simulink model "quadcopter_package_delivery"  (R2022a)
settings: Solver=ode23t  StartTime=0.0  StopTime=timespot_spl(end)+4  FixedStep=0.01  MaxStep=1e-2  RelTol=1e-3  AbsTol=1e-3
PostLoadFcn:
  | warning('off','sm:sli:setup:compile:LocalSolverNotSupported')
model workspace (MATLAB code in the model file):
  | load('xy_data_membrane.mat');
undefined symbols (not defined in the file): battery_capacity, filtD_altitude, filtD_attitude, filtD_motor, filtD_position, filtD_yaw, filtM_altitude, filtM_attitude, filtM_position, filtM_yaw, filtSpd_motor, kd_altitude, kd_attitude, kd_motor, kd_position, kd_yaw, ki_altitude, ki_attitude, ki_motor, ki_position, ki_yaw, kp_altitude, kp_attitude, kp_motor, kp_position, kp_yaw, limit_altitude, limit_attitude, limit_motor, limit_yaw, pkgDensity, planedepth, pos2attitude, qd_area, qd_drag, spline_data, spline_yaw, timespot_spl, waypoints, X, Y, Z
libraries: sm_lib x104, nesl_utility x61, fl_lib x21, slpidlib x9, ee_lib x5, quadcopter_library x4
(part 1 of 5)
CloseFcn:
  | try,close(h1_quadcopter_package_delivery),end
  | clear h1_quadcopter_package_delivery
  | try,close(h2_quadcopter_package_delivery),end
  | clear h2_quadcopter_package_delivery
  | try,close(h3_quadcopter_package_delivery),end
  | clear h3_quadcopter_package_delivery
  | try,close(h4_quadcopter_package_delivery),end
  | clear h4_quadcopter_package_delivery
Description:
  | Quadcopter Package Delivery
  | Copyright 2021 The MathWorks, Inc.
settings Model: Creator=tianwang  LastModifiedBy=johnsongash
settings SolverCC: AutoScaleAbsTol=off  AlgebraicLoopSolver=TrustRegion  SolverResetMethod=Robust
settings DataIOCC: MaxDataPoints=10000  ReturnWorkspaceOutputs=off  SignalLoggingName=logsout_quadcopter_package_delivery
settings DebuggingCC: ParameterPrecisionLossMsg=none  UnconnectedInputMsg=warning  UnconnectedOutputMsg=warning  UnconnectedLineMsg=warning  SFMachineParentedDataDiag=warning
settings SFSimCC: CustomCodeUndefinedFunction=UseInterfaceOnly
settings RTWCC: DLArmComputeVersion=19.05
settings SimscapeCC: ExplicitSolverDiagnosticOptions=none  SimscapeLogType=all  SimscapeLogSimulationStatistics=on  SimscapeLogToSDI=on  SimscapeLogName=simlog_quadcopter_package_delivery  SimscapeLogDataHistory=10000
settings DiagnosticsConfigSet: SimMechanicsConflictingReferenceFrames=none  SimMechanicsRigidlyBoundBlock=none
settings ExplorerConfigSet: InternalSimMechanicsExplorerSettings="<ExplorerConfiguration><canonicalview>default</canonicalview><AnimationSetting><BasePlaybackSpeed>1.0</BasePlaybackSpeed><PlaybackSpeedFactor>2.0</PlaybackSpeedFactor></AnimationSetting><TilePanel><TileInfo><Tiles Columns=\"2\" Count=\"4\" Rows=\"2\"><Column Weight=\"0.5664\"/><Column Weight=\"0.4336\"/><Row Weight=\"0.3531\"/><Row Weight=\"0.6469\"/><Tile Height=\"1\" Width=\"1\" X=\"0\" Y=\"0\"/><Tile Height=\"1\" Width=\"1\" X=\"0\" Y=\"1\"/><Tile Height=\"1\" Width=\"1\" X=\"1\" Y=\"0\"/><Tile Height=\"1\" Width=\"1\" X=\"1\" Y=\"1\"/></Tiles></TileInfo><SceneInfo><SceneViewer><BGColor><R>1</R><G>1</G><B>1</B></BGColor><Camera><DoPerspective>off</DoPerspective><Position><X>3.00027489530859626</X><Y>2.64492473252887361</Y><Z>13.644244441979108</Z></Position><Center><X>3.00027489530859626</X><Y>2.64492473252887361</Y><Z>3.00000062058594352</Z></Center><Up><X>0</X><Y>1</Y><Z>-0</Z></Up><ViewLimDist>1</ViewLimDist><YLim>10.5985457420349132</YLim><XLim>33.4261827248793395</XLim></Camera></SceneViewer><SceneViewer><BGColor><R>1</R><G>1</G><B>1</B></BGColor><Camera><DoPerspective>on</DoPerspective><Position><X>5.02017998369651863</X><Y>7.98844218227809488</Y><Z>3.70518563279751856</Z></Position><Center><X>5.02017998369651863</X><Y>7.98844218227809488</Y><Z>2.70518563279751856</Z></Center><Up><X>0</X><Y>1</Y><Z>0</Z></Up><ViewLimDist>1</ViewLimDist><YLim>0.466307658154998583</YLim><XLim>0.796608916014789226</XLim></Camera></SceneViewer><SceneViewer><BGColor><R>1</R><G>1</G><B>1</B></BGColor><Camera><DoPerspective>on</DoPerspective><Position><X>6.5</X><Y>6.5</Y><Z>1</Z></Position><Center><X>5</X><Y>8</Y><Z>0</Z></Center><Up><X>0</X><Y>0</Y><Z>1</Z></Up><ViewLimDist>1</ViewLimDist><YLim>0.466307658154998583</YLim><XLim>1.12272536155780434</XLim></Camera></SceneViewer><SceneViewer><BGColor><R>1</R><G>1</G><B>1</B></BGColor><Camera><DoPerspective>on</DoPerspective><Position><X>5.52017998369651863</X><Y>6.98844218227809488</Y><Z>3.70518563279751856</Z></Position><Center><X>5.1868466503631856</X><Y>7.65510884894476185</Y><Z>3.0385189661308516</Z></Center><Up><X>-0.298142396999971915</X><Y>0.596284793999944052</Y><Z>0.745355992499929787</Z></Up><ViewLimDist>1</ViewLimDist><YLim>0.466307658154998583</YLim><XLim>0.608142904177144006</XLim></Camera></SceneViewer></SceneInfo></TilePanel><MechEditorPanel><Cameras><Camera><Id>Camera1</Id><Value><Name>FixO Top</Name><NativeCamera><PositionTrackingFeature>Quadcopter.Camera.Cam_FixO_Top.R</PositionTrackingFeature><CenterTrackingFeature>Quadcopter.Camera.Cam_FixO_Top.R</CenterTrackingFeature><UpVectorTrackingFeature>Quadcopter.Camera.Cam_FixO_Top.R</UpVectorTrackingFeature><CenterTrackingOrigin>off</CenterTrackingOrigin><CenterTrackingDirection>+X</CenterTrackingDirection><UpVectorTrackingDirection>+Y</UpVectorTrackingDirection></NativeCamera></Value></Camera><Camera><Id>Camera2</Id><Value><Name>FixO L</Name><NativeCamera><PositionTrackingFeature>Quadcopter.Camera.Cam_FixO_L.R</PositionTrackingFeature><CenterTrackingFeature>Quadcopter.Camera.Cam_FixO_L.R</CenterTrackingFeature><UpVectorTrackingFeature>Quadcopter.Camera.Cam_FixO_L.R</UpVectorTrackingFeature><CenterTrackingOrigin>off</CenterTrackingOrigin><CenterTrackingDirection>+X</CenterTrackingDirection><UpVectorTrackingDirection>+Z</UpVectorTrackingDirection></NativeCamera></Value></Camera><Camera><Id>Camera3</Id><Value><Name>FixO F</Name><NativeCamera><PositionTrackingFeature>Quadcopter.Camera.Cam_FixO_F.R</PositionTrackingFeature><CenterTrackingFeature>Quadcopter.Camera.Cam_FixO_F.R</CenterTrackingFeature><UpVectorTrackingFeature>Quadcopter.Camera.Cam_FixO_F.R</UpVectorTrackingFeature><CenterTrackingOrigin>off</CenterTrackingOrigin><CenterTrackingDirection>+X</CenterTrackingDirection><UpVectorTrackingDirection>+Z</UpVectorTrackingDirection></NativeCamera></Value></Camera><Camera><Id>Camera4</Id><Value><Name>FixO UFL</Name><NativeCamera><PositionTrackingFeature>Quadcopter.Camera.Cam_FixO_UFL.R</PositionTrackingFeature><CenterTrackingFeature>Quadcopter.Camera.Cam_FixO_UFL.R</CenterTrackingFeature><UpVectorTrackingFeature>Quadcopter.Camera.Cam_FixO_UFL.R</UpVectorTrackingFeature><CenterTrackingOrigin>off</CenterTrackingOrigin><CenterTrackingDirection>+X</CenterTrackingDirection><UpVectorTrackingDirection>+Z</UpVectorTrackingDirection></NativeCamera></Value></Camera><Camera><Id>Camera5</Id><Value><Name>Track_Target</Name><NativeCamera><PositionTrackingFeature>Quadcopter.Camera.Cam_Target.R</PositionTrackingFeature><CenterTrackingFeature>Quadcopter.Camera.Transform_Target.F</CenterTrackingFeature><UpVectorTrackingFeature>Quadcopter.Camera.Transform_Target.F</UpVectorTrackingFeature><CenterTrackingOrigin>on</CenterTrackingOrigin><UpVectorTrackingDirection>+Z</UpVectorTrackingDirection></NativeCamera></Value></Camera><Camera><Id>Camera6</Id><Value><Name>Track Body Forward</Name><NativeCamera><PositionTrackingFeature>Quadcopter.Body.Body.Cam_Body_Front.R</PositionTrackingFeature><CenterTrackingFeature>Quadcopter.Body.Body.Cam_Body_Front.R</CenterTrackingFeature><UpVectorTrackingFeature>Quadcopter.Body.Body.Cam_Body_Front.R</UpVectorTrackingFeature><CenterTrackingOrigin>off</CenterTrackingOrigin><CenterTrackingDirection>+X</CenterTrackingDirection><UpVectorTrackingDirection>+Z</UpVectorTrackingDirection></NativeCamera></Value></Camera></Cameras><GfxPanelCameraMap><MapElement CameraMLId=\"Camera1\" GfxPanelIndex=\"1\"/><MapElement CameraMLId=\"Camera5\" GfxPanelIndex=\"2\"/><MapElement CameraMLId=\"Camera4\" GfxPanelIndex=\"3\"/></GfxPanelCameraMap><VideoCreator><PlaybackSpeedRatio>1.0</PlaybackSpeedRatio><FrameRate>60</FrameRate><VideoFormat>MPEG-4</VideoFormat><FrameSize>[1920 1080]</FrameSize></VideoCreator></MechEditorPanel></ExplorerConfiguration>"

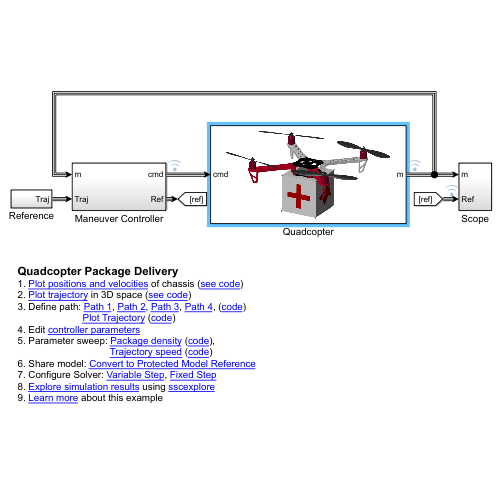
[thumbnail: Simulink's stored preview of the top-level diagram]
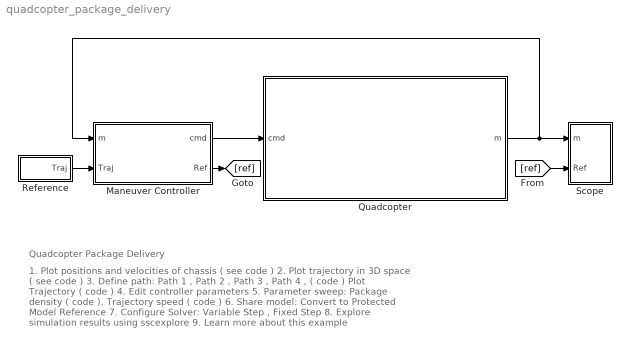
== system quadcopter_package_delivery ==
  note: Quadcopter Package Delivery
  note: 1. Plot positions and velocities of chassis ( see code )
      | 2. Plot trajectory in 3D space ( see code )
      | 3. Define path: Path 1 , Path 2 , Path 3 , Path 4 , ( code )
      | Plot Trajectory ( code )
      | 4. Edit controller parameters
      | 5. Parameter sweep: Package density ( code ),
      | Trajectory speed ( code )
      | 6. Share model: Convert to Protected Model Reference
      | 7. Configure Solver: Variable Step , Fixed Step
      | 8. Explore simulation results using sscexplore
      | 9. Learn more about this example
  Maneuver Controller : Subsystem
  Quadcopter : Subsystem
      mask Display: image('quadcopter_body_arms_load.png');
  Reference : Subsystem
  Scope : Subsystem
  wires:
  Maneuver Controller/1(cmd) -> Quadcopter/1(cmd)
  Quadcopter/1(m) -> Scope/1(m), Maneuver Controller/1(m)
  Reference/1(Traj) -> Maneuver Controller/2(Traj)
  [ref] -> Scope/2(Ref)
  Maneuver Controller/2(Ref) -> [ref]

== system quadcopter_package_delivery/Maneuver Controller ==
  In Bus Element13 : Inport  PortName=m
  In Bus Element3 : Inport  Port=2  PortName=Traj
  Altitude and YPR Control : Subsystem  mask{attitude_filtM=filtM_attitude, attitude_kp=kp_attitude, attitude_ki=ki_attitude, attitude_kd=kd_attitude, attitude_f=filtD_attitude, attitude_limit=limit_attitude, yaw_filtM=filtM_yaw, yaw_kp=kp_yaw, yaw_ki=ki_yaw, yaw_kd=kd_yaw, yaw_f=filtD_yaw, yaw_limit=limit_yaw, altitude_filtM=filtM_altitude, altitude_kp=kp_altitude, altitude_ki=ki_altitude, altitude_kd=kd_altitude, altitude_f=filtD_altitude, altitude_limit=limit_altitude}
      mask prompts: attitude_filtM "Filter Measurement (s)"; attitude_kp "Kp"; attitude_ki "Ki"; attitude_kd "Kd"; attitude_f "Derivative Filter Coefficient"; attitude_limit "Limit (m/s)"; yaw_filtM "Filter Measurement (s)"; yaw_kp "Kp"; yaw_ki "Ki"; yaw_kd "Kd"; yaw_f "Derivative Filter Coefficient"; yaw_limit "Limit (m/s)"; altitude_filtM "Filter Measurement (s)"; altitude_kp "Kp"; altitude_ki "Ki"; altitude_kd "Kd"; altitude_f "Derivative Filter Coefficient"; altitude_limit "Limit (m/s)"
      mask DialogControl Container3 Prompt: Attitude (Orientation)
      mask DialogControl Container4 Prompt: Yaw
      mask DialogControl Container_alt Prompt: Altitude (Orientation)
  Motor Mixer : Subsystem
  Position Control : Subsystem  mask{filt_pos4attitude=filtM_position, kp_xy2ypr=kp_position, ki_xy2ypr=ki_position, kd_xy2ypr=kd_position, filtD_xy2ypr=filtD_position, err2rp=pos2attitude}
      mask prompts: filt_pos4attitude "Filter Constant (s)"; kp_xy2ypr "Kp"; ki_xy2ypr "Ki"; kd_xy2ypr "Kd"; filtD_xy2ypr "Derivative Filter Coefficient"; err2rp "Position Error to Attitude"
  cmd : Outport
  Ref : Outport  Port=2
  wires:
  Motor Mixer/1(Cmd) -> cmd/1
  Altitude and YPR Control/2(Motor Roll) -> Motor Mixer/2(Roll Cmd)
  Altitude and YPR Control/1(Motor Pitch) -> Motor Mixer/1(Pitch Cmd)
  Altitude and YPR Control/3(Motor Yaw) -> Motor Mixer/3(Yaw Cmd)
  Altitude and YPR Control/4(Motor Thrust) -> Motor Mixer/4(Thrust Cmd)
  Position Control/2(Roll Cmd) -> Altitude and YPR Control/4(Roll Cmd)
  Position Control/1(Pitch Cmd) -> Altitude and YPR Control/3(Pitch Cmd)
  In Bus Element13/1 -> Position Control/1(m), Altitude and YPR Control/1(m)
  In Bus Element3/1 -> Position Control/2(Traj), Altitude and YPR Control/2(Ref)
  Position Control/3(Yaw Cmd) -> Altitude and YPR Control/5(Yaw Cmd)
  Position Control/4(Ref) -> Ref/1

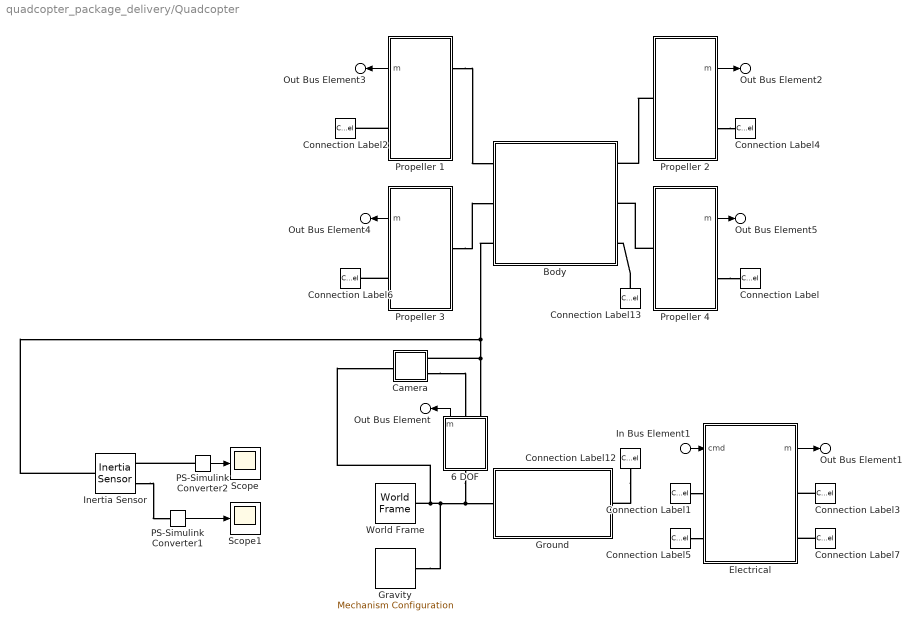
== system quadcopter_package_delivery/Quadcopter ==
  In Bus Element1 : Inport  PortName=cmd
  6 DOF : Subsystem
  Body : Subsystem
      mask Display: image('quadcopter_body_arms.png');
  Camera : Subsystem
  Connection Label : ConnectionLabel  Label=P4
  Connection Label1 : ConnectionLabel  Label=P4
  Connection Label12 : ConnectionLabel  Label=G
  Connection Label13 : ConnectionLabel  Label=G
  Connection Label2 : ConnectionLabel  Label=P1
  Connection Label3 : ConnectionLabel  Label=P1
  Connection Label4 : ConnectionLabel  Label=P2
  Connection Label5 : ConnectionLabel  Label=P2
  Connection Label6 : ConnectionLabel  Label=P3
  Connection Label7 : ConnectionLabel  Label=P3
  Electrical : Subsystem  mask{trq_max=0.8, power_max=80, trq_tc=0.02, eff_overall=25/30*100, eff_spd=5000, eff_trq=0.05, rotor_d=1e-7, kp=kp_motor, ki=ki_motor, kd=kd_motor, f_deriv=filtD_motor, f_spd=filtSpd_motor, max_trq_cmd=limit_motor}
      mask prompts: trq_max "Max Torque (N*m)"; power_max "Max Power (W)"; trq_tc "Time Constant, Torque (s)"; eff_overall "Efficiency (%)"; eff_spd "Speed for Efficiency (rpm)"; eff_trq "Torque for Efficiency (N*m)"; rotor_d "Rotor Damping (N*m/(rad/s))"; kp "Proportional"; ki "Integral"; kd "Derivative"; f_deriv "Filter on Error Derivative (N)"; f_spd "Filter on Speed Measurement (sec)"; max_trq_cmd "Saturation (N*m)"
      mask DialogControl Container4 Prompt: Motor
      mask DialogControl Container9 Prompt: Control
      mask Display: image('quadcopter_electric.png');
  Gravity : sm_lib/Utilities/Mechanism Configuration  UniformGravity=Constant  GravityVector=[0 0 -9.80665]  GravityUnits=m/s^2  LinearizationDelta=0.001  JointModeTransitionNonlinearIterations=2
  Ground : Subsystem
      mask Display: image('ground_launch_target.PNG');
  Inertia Sensor : sm_lib/Body Elements/Inertia Sensor  SensorExtent=BodyGroup  SpanWeldJoints=off  ExcludeGroundedBodies=off  MeasurementFrame=Attached  SenseMass=on  SenseCenterOfMass=off  SenseInertiaMatrix=on  SenseCenteredInertiaMatrix=off  SensePrincipalInertiaMatrix=off  SenseRotationMatrix=off  GraphicType=PrincipalInertiaFrame  PrincipalInertiaFrameSize=20  GraphicVisPropType=SimpleVisualProperties  GraphicDiffuseColor=[0.5 0.5 0.5]  GraphicSpecularColor=[0.5 0.5 0.5 1.0]  GraphicAmbientColor=[0.15 0.15 0.15 1.0]  GraphicEmissiveColor=[0.0 0.0 0.0 1.0]  GraphicShininess=75  GraphicOpacity=1.0
      settings: SourceProductBaseCode=MS
  PS-Simulink Converter1 : nesl_utility/PS-Simulink Converter  PhysicalDomain=network_engine_domain  SubClassName=ps_output  LeftPortType=input  RightPortType=output  PseudoPeriodic=off  Frequencies=[]  VectorFormat=inherit  Unit=inherit  AffineConversion=off
      settings: SourceProductBaseCode=SS,PW,VE
  PS-Simulink Converter2 : nesl_utility/PS-Simulink Converter  PhysicalDomain=network_engine_domain  SubClassName=ps_output  LeftPortType=input  RightPortType=output  PseudoPeriodic=off  Frequencies=[]  VectorFormat=inherit  Unit=inherit  AffineConversion=off
      settings: SourceProductBaseCode=SS,PW,VE
  Propeller 1 : Subsystem  AncestorBlock=quadcopter_library/Propeller  mask{popup_prop_pos=1 or 4}
      mask prompts: popup_prop_pos "Propeller Position"
      mask init:
      | if(strcmp(get_param(gcb,'popup_prop_pos'),'1 or 4'))
      |     set_param([gcb '/Propeller'],'ExtGeomFileName','quadcopter_drone_propeller_1_4.stp');
      | else
      |     set_param([gcb '/Propeller'],'ExtGeomFileName','quadcopter_drone_propeller_2_3.stp');
      | end
      mask TypeOptions popup_prop_pos: 1 or 4 | 2 or 3
      mask Display:
      | if(strcmp(get_param(gcb,'popup_prop_pos'),'1 or 4'))
      |     image('quadcopter_motor_prop_1_4.png');
      | else
      |     image('quadcopter_motor_prop_2_3.png');
      | end
  Propeller 2 : Subsystem  AncestorBlock=quadcopter_library/Propeller  mask{popup_prop_pos=2 or 3}
      mask prompts: popup_prop_pos "Propeller Position"
      mask init: same as quadcopter_package_delivery/Quadcopter/Propeller 1
      mask TypeOptions popup_prop_pos: 1 or 4 | 2 or 3
      mask Display:
      | if(strcmp(get_param(gcb,'popup_prop_pos'),'1 or 4'))
      |     image('quadcopter_motor_prop_1_4.png');
      | else
      |     image('quadcopter_motor_prop_2_3.png');
      | end
  Propeller 3 : Subsystem  AncestorBlock=quadcopter_library/Propeller  mask{popup_prop_pos=2 or 3}
      mask prompts: popup_prop_pos "Propeller Position"
      mask init: same as quadcopter_package_delivery/Quadcopter/Propeller 1
      mask TypeOptions popup_prop_pos: 1 or 4 | 2 or 3
      mask Display:
      | if(strcmp(get_param(gcb,'popup_prop_pos'),'1 or 4'))
      |     image('quadcopter_motor_prop_1_4.png');
      | else
      |     image('quadcopter_motor_prop_2_3.png');
      | end
  Propeller 4 : Subsystem  AncestorBlock=quadcopter_library/Propeller  mask{popup_prop_pos=1 or 4}
      mask prompts: popup_prop_pos "Propeller Position"
      mask init: same as quadcopter_package_delivery/Quadcopter/Propeller 1
      mask TypeOptions popup_prop_pos: 1 or 4 | 2 or 3
      mask Display:
      | if(strcmp(get_param(gcb,'popup_prop_pos'),'1 or 4'))
      |     image('quadcopter_motor_prop_1_4.png');
      | else
      |     image('quadcopter_motor_prop_2_3.png');
      | end
  Scope : Scope
  Scope1 : Scope
  World Frame : sm_lib/Frames and Transforms/World Frame
  Out Bus Element : Outport  PortName=m  Element=Chassis
  Out Bus Element1 : Outport  PortName=m  Element=Motor
  Out Bus Element2 : Outport  PortName=m  Element=Prop2
  Out Bus Element3 : Outport  PortName=m  Element=Prop1
  Out Bus Element4 : Outport  PortName=m  Element=Prop3
  Out Bus Element5 : Outport  PortName=m  Element=Prop4
  wires:
  Propeller 4/1(m) -> Out Bus Element5/1
  Propeller 1/1(m) -> Out Bus Element3/1
  Propeller 3/1(m) -> Out Bus Element4/1
  Electrical/1(m) -> Out Bus Element1/1
  Propeller 2/1(m) -> Out Bus Element2/1
  In Bus Element1/1 -> Electrical/1(cmd)
  6 DOF/1(m) -> Out Bus Element/1
  PS-Simulink Converter1/1 -> Scope1/1
  PS-Simulink Converter2/1 -> Scope/1
  connections:
  Body/LConn3 -- Inertia Sensor/LConn1 -- 6 DOF/RConn2 -- Camera/RConn1
  Propeller 2/LConn1 -- Body/RConn1
  Propeller 1/LConn1 -- Body/LConn1
  Propeller 4/LConn1 -- Body/RConn2
  Propeller 3/LConn1 -- Body/LConn2
  Connection Label13/LConn1 -- Body/RConn3
  Propeller 4/RConn1 -- Connection Label/LConn1
  Connection Label1/LConn1 -- Electrical/LConn1
  Propeller 1/RConn1 -- Connection Label2/LConn1
  Connection Label3/LConn1 -- Electrical/RConn1
  Propeller 2/RConn1 -- Connection Label4/LConn1
  Connection Label5/LConn1 -- Electrical/LConn2
  Propeller 3/RConn1 -- Connection Label6/LConn1
  Connection Label7/LConn1 -- Electrical/RConn2
  Gravity/RConn1 -- Camera/LConn1 -- World Frame/RConn1 -- Ground/RConn1 -- 6 DOF/LConn1
  Connection Label12/LConn1 -- Ground/LConn1
  Camera/RConn2 -- 6 DOF/RConn1
  Inertia Sensor/RConn2 -- PS-Simulink Converter1/LConn1
  PS-Simulink Converter2/LConn1 -- Inertia Sensor/RConn1

== system quadcopter_package_delivery/Reference ==
  Clock1 : Clock
  Derivative : Subsystem
  Derivative1 : Subsystem
  Interpolate Spline Points : Subsystem
  Out Bus Element : Outport  PortName=Traj  Element=pos
  Out Bus Element1 : Outport  PortName=Traj  Element=vel
  Out Bus Element2 : Outport  PortName=Traj  Element=yaw
  Out Bus Element3 : Outport  PortName=Traj  Element=acc
  wires:
  Clock1/1 -> Interpolate Spline Points/1(In1)
  Interpolate Spline Points/2(des_pos) -> Out Bus Element/1, Derivative/1(des xyz)
  Interpolate Spline Points/1(Yaw) -> Out Bus Element2/1
  Derivative/1(des_vel) -> Derivative1/1(des vel), Out Bus Element1/1
  Derivative1/1(des_acc) -> Out Bus Element3/1

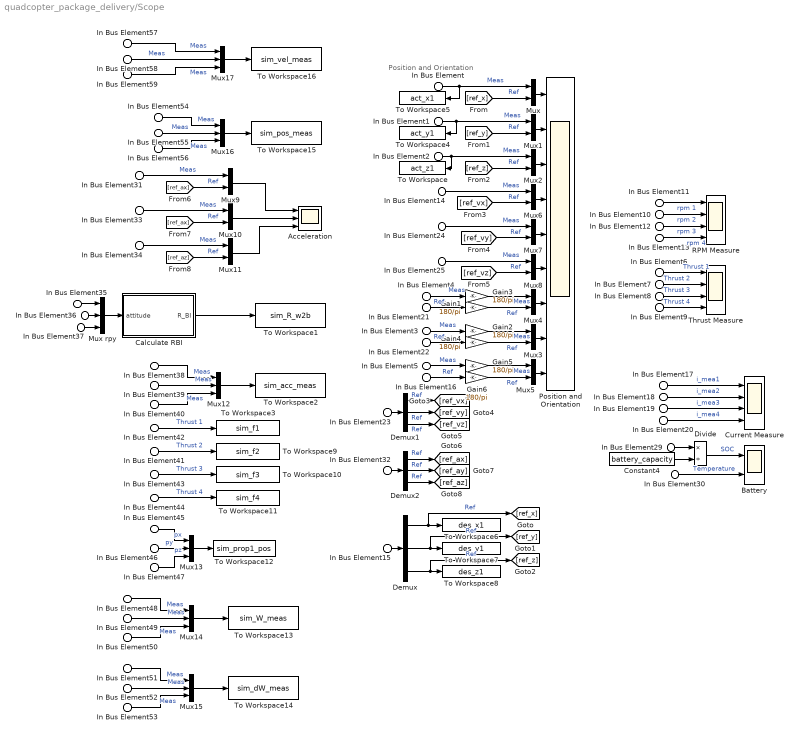
== system quadcopter_package_delivery/Scope ==
  note: Position and Orientation
  In Bus Element : Inport  PortName=m  Element=Chassis.px
  In Bus Element54 : Inport  PortName=m  Element=Chassis.px
  In Bus Element1 : Inport  PortName=m  Element=Chassis.py
  In Bus Element55 : Inport  PortName=m  Element=Chassis.py
  In Bus Element2 : Inport  PortName=m  Element=Chassis.pz
  In Bus Element56 : Inport  PortName=m  Element=Chassis.pz
  In Bus Element3 : Inport  PortName=m  Element=Chassis.pitch
  In Bus Element36 : Inport  PortName=m  Element=Chassis.pitch
  In Bus Element4 : Inport  PortName=m  Element=Chassis.roll
  In Bus Element35 : Inport  PortName=m  Element=Chassis.roll
  In Bus Element5 : Inport  PortName=m  Element=Chassis.yaw
  In Bus Element37 : Inport  PortName=m  Element=Chassis.yaw
  In Bus Element14 : Inport  PortName=m  Element=Chassis.vx
  In Bus Element57 : Inport  PortName=m  Element=Chassis.vx
  In Bus Element24 : Inport  PortName=m  Element=Chassis.vy
  In Bus Element58 : Inport  PortName=m  Element=Chassis.vy
  In Bus Element25 : Inport  PortName=m  Element=Chassis.vz
  In Bus Element59 : Inport  PortName=m  Element=Chassis.vz
  In Bus Element31 : Inport  PortName=m  Element=Chassis.ax
  In Bus Element38 : Inport  PortName=m  Element=Chassis.ax
  In Bus Element33 : Inport  PortName=m  Element=Chassis.ay
  In Bus Element39 : Inport  PortName=m  Element=Chassis.ay
  In Bus Element34 : Inport  PortName=m  Element=Chassis.az
  In Bus Element40 : Inport  PortName=m  Element=Chassis.az
  In Bus Element48 : Inport  PortName=m  Element=Chassis.wx
  In Bus Element49 : Inport  PortName=m  Element=Chassis.wy
  In Bus Element50 : Inport  PortName=m  Element=Chassis.wz
  In Bus Element51 : Inport  PortName=m  Element=Chassis.dwx
  In Bus Element52 : Inport  PortName=m  Element=Chassis.dwy
  In Bus Element53 : Inport  PortName=m  Element=Chassis.dwz
  In Bus Element7 : Inport  PortName=m  Element=Prop2.thrust
  In Bus Element41 : Inport  PortName=m  Element=Prop2.thrust
  In Bus Element10 : Inport  PortName=m  Element=Prop2.w
  In Bus Element6 : Inport  PortName=m  Element=Prop1.thrust
  In Bus Element42 : Inport  PortName=m  Element=Prop1.thrust
  In Bus Element11 : Inport  PortName=m  Element=Prop1.w
  In Bus Element45 : Inport  PortName=m  Element=Prop1.px
  In Bus Element46 : Inport  PortName=m  Element=Prop1.py
  In Bus Element47 : Inport  PortName=m  Element=Prop1.pz
  In Bus Element8 : Inport  PortName=m  Element=Prop3.thrust
  In Bus Element43 : Inport  PortName=m  Element=Prop3.thrust
  In Bus Element12 : Inport  PortName=m  Element=Prop3.w
  In Bus Element9 : Inport  PortName=m  Element=Prop4.thrust
  In Bus Element44 : Inport  PortName=m  Element=Prop4.thrust
  In Bus Element13 : Inport  PortName=m  Element=Prop4.w
  In Bus Element17 : Inport  PortName=m  Element=Motor.Mot1.i
  In Bus Element18 : Inport  PortName=m  Element=Motor.Mot2.i
  In Bus Element19 : Inport  PortName=m  Element=Motor.Mot3.i
  In Bus Element20 : Inport  PortName=m  Element=Motor.Mot4.i
  In Bus Element29 : Inport  PortName=m  Element=Motor.Battery.SOC
  In Bus Element30 : Inport  PortName=m  Element=Motor.Battery.degC
  In Bus Element15 : Inport  Port=2  PortName=Ref  Element=pos
  In Bus Element16 : Inport  Port=2  PortName=Ref  Element=yaw
  In Bus Element21 : Inport  Port=2  PortName=Ref  Element=roll
  In Bus Element22 : Inport  Port=2  PortName=Ref  Element=pitch
  In Bus Element23 : Inport  Port=2  PortName=Ref  Element=vel
  In Bus Element32 : Inport  Port=2  PortName=Ref  Element=acc
  Acceleration : Scope  NumInputPorts=3
  Battery : Scope  NumInputPorts=2
  Calculate RBI : MATLAB Function  TreatAsAtomicUnit=on
  Constant4 : Constant  Value=battery_capacity
  Current Measure : Scope  NumInputPorts=4
  Demux : Demux  Outputs=3
  Demux1 : Demux  Outputs=3
  Demux2 : Demux  Outputs=3
  Divide : Product  Inputs=*/
  Gain{1..6} (6 alike) : Gain  Gain=180/pi
  Mux{,1..11} (12 alike) : Mux  Inputs=2
  Mux rpy : Mux  Inputs=3
  Mux{12..17} (6 alike) : Mux  Inputs=3
  Position and Orientation : Scope  NumInputPorts=9
  RPM Measure : Scope  NumInputPorts=4
  Thrust Measure : Scope  NumInputPorts=4
  To Workspace : ToWorkspace  VariableName=act_z1  SampleTime=-1
  To Workspace1 : ToWorkspace  VariableName=sim_R_w2b  SaveFormat=Structure With Time  SampleTime=-1
  To Workspace10 : ToWorkspace  VariableName=sim_f3  SaveFormat=Structure With Time  SampleTime=-1
  To Workspace11 : ToWorkspace  VariableName=sim_f4  SaveFormat=Structure With Time  SampleTime=-1
  To Workspace12 : ToWorkspace  VariableName=sim_prop1_pos  SaveFormat=Structure With Time  SampleTime=-1
  To Workspace13 : ToWorkspace  VariableName=sim_W_meas  SaveFormat=Structure With Time  SampleTime=-1
  To Workspace14 : ToWorkspace  VariableName=sim_dW_meas  SaveFormat=Structure With Time  SampleTime=-1
  To Workspace15 : ToWorkspace  VariableName=sim_pos_meas  SaveFormat=Structure With Time  SampleTime=-1
  To Workspace16 : ToWorkspace  VariableName=sim_vel_meas  SaveFormat=Structure With Time  SampleTime=-1
  To Workspace2 : ToWorkspace  VariableName=sim_acc_meas  SaveFormat=Structure With Time  SampleTime=-1
  To Workspace3 : ToWorkspace  VariableName=sim_f1  SaveFormat=Structure With Time  SampleTime=-1
  To Workspace4 : ToWorkspace  VariableName=act_y1  SampleTime=-1
  To Workspace5 : ToWorkspace  VariableName=act_x1  SampleTime=-1
  To Workspace6 : ToWorkspace  VariableName=des_x1  SampleTime=-1
  To Workspace7 : ToWorkspace  VariableName=des_y1  SampleTime=-1
  To Workspace8 : ToWorkspace  VariableName=des_z1  SampleTime=-1
  To Workspace9 : ToWorkspace  VariableName=sim_f2  SaveFormat=Structure With Time  SampleTime=-1
  wires:
  In Bus Element7/1 -> Thrust Measure/2  "Thrust 2"
  In Bus Element9/1 -> Thrust Measure/4  "Thrust 4"
  In Bus Element8/1 -> Thrust Measure/3  "Thrust 3"
  In Bus Element6/1 -> Thrust Measure/1  "Thrust 1"
  In Bus Element11/1 -> RPM Measure/1  "rpm 1"
  In Bus Element10/1 -> RPM Measure/2  "rpm 2"
  In Bus Element12/1 -> RPM Measure/3  "rpm 3"
  In Bus Element13/1 -> RPM Measure/4  "rpm 4"
  Demux/3 -> [ref_z], To Workspace8/1  "Ref"
  In Bus Element2/1 -> Mux2/1, To Workspace/1  "Meas"
  In Bus Element17/1 -> Current Measure/1  "i_mea1"
  In Bus Element18/1 -> Current Measure/2  "i_mea2"
  In Bus Element19/1 -> Current Measure/3  "i_mea3"
  In Bus Element20/1 -> Current Measure/4  "i_mea4"
  Gain2/1 -> Mux3/1  "Meas"
  Gain3/1 -> Mux4/1  "Meas"
  Gain5/1 -> Mux5/1  "Meas"
  Demux/2 -> [ref_y], To Workspace7/1  "Ref"
  In Bus Element1/1 -> Mux1/1, To Workspace4/1  "Meas"
  Demux/1 -> To Workspace6/1, [ref_x]  "Ref"
  In Bus Element/1 -> Mux/1, To Workspace5/1  "Meas"
  Mux/1 -> Position and Orientation/1
  Mux1/1 -> Position and Orientation/2
  Mux2/1 -> Position and Orientation/3
  Mux3/1 -> Position and Orientation/8
  Mux4/1 -> Position and Orientation/7
  Mux5/1 -> Position and Orientation/9
  In Bus Element15/1 -> Demux/1
  [ref_x] -> Mux/2  "Ref"
  [ref_y] -> Mux1/2  "Ref"
  [ref_z] -> Mux2/2  "Ref"
  In Bus Element23/1 -> Demux1/1
  Demux1/1 -> [ref_vx]  "Ref"
  Demux1/2 -> [ref_vy]  "Ref"
  Demux1/3 -> [ref_vz]  "Ref"
  Mux8/1 -> Position and Orientation/6
  Mux7/1 -> Position and Orientation/5
  Mux6/1 -> Position and Orientation/4
  [ref_vx] -> Mux6/2  "Ref"
  [ref_vy] -> Mux7/2  "Ref"
  [ref_vz] -> Mux8/2  "Ref"
  In Bus Element14/1 -> Mux6/1  "Meas"
  In Bus Element24/1 -> Mux7/1  "Meas"
  In Bus Element25/1 -> Mux8/1  "Meas"
  In Bus Element21/1 -> Gain1/1  "Ref"
  In Bus Element22/1 -> Gain4/1  "Ref"
  In Bus Element16/1 -> Gain6/1  "Ref"
  In Bus Element4/1 -> Gain3/1  "Meas"
  Gain1/1 -> Mux4/2  "Ref"
  In Bus Element3/1 -> Gain2/1  "Meas"
  Gain4/1 -> Mux3/2  "Ref"
  In Bus Element5/1 -> Gain5/1  "Meas"
  Gain6/1 -> Mux5/2  "Ref"
  In Bus Element29/1 -> Divide/1
  Constant4/1 -> Divide/2
  Divide/1 -> Battery/1  "SOC"
  In Bus Element30/1 -> Battery/2  "Temperature"
  In Bus Element31/1 -> Mux9/1  "Meas"
  [ref_ax] -> Mux9/2  "Ref"
  In Bus Element32/1 -> Demux2/1
  Demux2/3 -> [ref_az]  "Ref"
  Demux2/1 -> [ref_ax]  "Ref"
  Demux2/2 -> [ref_ay]  "Ref"
  Mux9/1 -> Acceleration/1
  [ref_ax] -> Mux10/2  "Ref"
  In Bus Element33/1 -> Mux10/1  "Meas"
  Mux10/1 -> Acceleration/2
  [ref_az] -> Mux11/2  "Ref"
  In Bus Element34/1 -> Mux11/1  "Meas"
  Mux11/1 -> Acceleration/3
  In Bus Element36/1 -> Mux rpy/2
  In Bus Element37/1 -> Mux rpy/3
  In Bus Element35/1 -> Mux rpy/1
  Mux rpy/1 -> Calculate RBI/1(attitude)
  Calculate RBI/1(R_BI) -> To Workspace1/1
  In Bus Element39/1 -> Mux12/2  "Meas"
  In Bus Element38/1 -> Mux12/1  "Meas"
  In Bus Element40/1 -> Mux12/3  "Meas"
  Mux12/1 -> To Workspace2/1
  In Bus Element42/1 -> To Workspace3/1  "Thrust 1"
  In Bus Element41/1 -> To Workspace9/1  "Thrust 2"
  In Bus Element43/1 -> To Workspace10/1  "Thrust 3"
  In Bus Element44/1 -> To Workspace11/1  "Thrust 4"
  Mux13/1 -> To Workspace12/1
  In Bus Element45/1 -> Mux13/1  "px"
  In Bus Element46/1 -> Mux13/2  "py"
  In Bus Element47/1 -> Mux13/3  "pz"
  In Bus Element50/1 -> Mux14/3  "Meas"
  In Bus Element48/1 -> Mux14/1  "Meas"
  In Bus Element49/1 -> Mux14/2  "Meas"
  Mux14/1 -> To Workspace13/1
  In Bus Element51/1 -> Mux15/1  "Meas"
  Mux15/1 -> To Workspace14/1
  In Bus Element53/1 -> Mux15/3  "Meas"
  In Bus Element52/1 -> Mux15/2  "Meas"
  In Bus Element55/1 -> Mux16/2  "Meas"
  In Bus Element54/1 -> Mux16/1  "Meas"
  In Bus Element56/1 -> Mux16/3  "Meas"
  Mux16/1 -> To Workspace15/1
  In Bus Element58/1 -> Mux17/2  "Meas"
  In Bus Element57/1 -> Mux17/1  "Meas"
  In Bus Element59/1 -> Mux17/3  "Meas"
  Mux17/1 -> To Workspace16/1

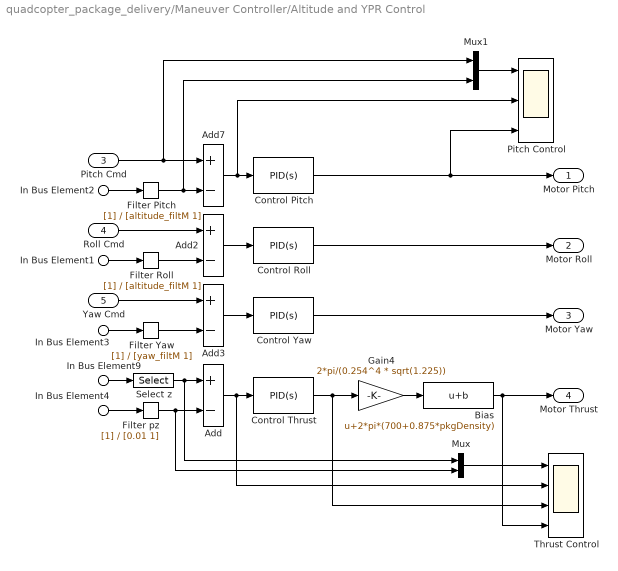
== system quadcopter_package_delivery/Maneuver Controller/Altitude and YPR Control ==
  In Bus Element1 : Inport  PortName=m  Element=Chassis.roll
  In Bus Element2 : Inport  PortName=m  Element=Chassis.pitch
  In Bus Element3 : Inport  PortName=m  Element=Chassis.yaw
  In Bus Element4 : Inport  PortName=m  Element=Chassis.pz
  In Bus Element9 : Inport  Port=2  PortName=Ref  Element=pos
  Pitch Cmd : Inport  Port=3
  Roll Cmd : Inport  Port=4
  Yaw Cmd : Inport  Port=5
  Add{,2..3,7} (4 alike) : Sum  Inputs=+-
  Bias : Bias  Bias=2*pi*(700+0.875*pkgDensity)  SaturateOnIntegerOverflow=off
  Control Pitch : slpidlib/PID Controller  Controller=PID  Form=Parallel  TimeDomain=Continuous-time  UseExternalTs=off  SampleTime=-1  IntegratorMethod=Forward Euler  FilterMethod=Forward Euler  ControllerParametersSource=internal  P=attitude_kp  I=attitude_ki  UseKiTs=off  D=attitude_kd  N=attitude_f  UseFilter=on  TunerSelectOption=Transfer Function Based (PID Tuner App)  InitialConditionSource=internal  InitialConditionForIntegrator=0  InitialConditionForFilter=0  DifferentiatorICPrevScaledInput=0  ExternalReset=none  TrackingMode=off  Kt=1  LimitOutput=on  SatLimitsSource=internal  UpperSaturationLimit=attitude_limit  LowerSaturationLimit=-attitude_limit  LinearizeAsGain=on  AntiWindupMode=none  Kb=1  POutMin=[]  POutMax=[]  IOutMin=[]  IOutMax=[]  DOutMin=[]  DOutMax=[]  NOutMin=[]  NOutMax=[]  SumOutMin=[]  SumOutMax=[]  SaturationOutMin=[]  SaturationOutMax=[]  PParamMin=[]  PParamMax=[]  IParamMin=[]  IParamMax=[]  DParamMin=[]  DParamMax=[]  NParamMin=[]  NParamMax=[]  KbParamMin=[]  KbParamMax=[]  KtParamMin=[]  KtParamMax=[]  KbOutMin=[]  KbOutMax=[]  KtOutMin=[]  KtOutMax=[]  IntegratorOutMin=[]  IntegratorOutMax=[]  FilterOutMin=[]  FilterOutMax=[]  SumI1OutMin=[]  SumI1OutMax=[]  SumI2OutMin=[]  SumI2OutMax=[]  SumI3OutMin=[]  SumI3OutMax=[]  SumI4OutMin=[]  SumI4OutMax=[]  SumDOutMin=[]  SumDOutMax=[]  DifferentiatorOutMin=[]  DifferentiatorOutMax=[]  FilterDiffOutCoefMin=[]  FilterDiffOutCoefMax=[]  ReciprocalOutMin=[]  ReciprocalOutMax=[]  SumDenOutMin=[]  SumDenOutMax=[]  SumNumOutMin=[]  SumNumOutMax=[]  DivideOutMin=[]  DivideOutMax=[]  UdiffTsProdOutMin=[]  UdiffTsProdOutMax=[]  NTsProdOutMin=[]  NTsProdOutMax=[]  UintegralTsProdOutMin=[]  UintegralTsProdOutMax=[]  UngainTsProdOutMin=[]  UngainTsProdOutMax=[]  IntegratorContinuousStateAttributes=''  IntegratorStateMustResolveToSignalObject=off  IntegratorRTWStateStorageClass=Auto  FilterContinuousStateAttributes=''  FilterStateMustResolveToSignalObject=off  FilterRTWStateStorageClass=Auto  ParallelPVariant=InternalParameters  IdealPVariant=Disabled  IVariant=InternalParameters  DVariant=InternalParameters  IntegratorVariant=Continuous  SatVariant=Enabled  AWVariant=Passthrough  PCopyVariant=Disabled  TRVariant=Disabled  FdbkBlocksVariant=Forward  IdealPFdbkVariant=Disabled  SatFdbkVariant=Disabled  DerivativeFilterVariant=ContFilter  NVariant=InternalParameters  NCopyVariant=Disabled  FilterICVariant=InternalICsFilter  IntegratorICVariant=InternalICs  ExternalResetVariant=Disabled  TRSumVariant=Passthrough  SumFdbkVariant=Disabled  SumVariant=Sum_PID  TsampFilterVariant=InternalTs  TsampNgainVariant=Passthrough  TsampIntegralVariant=Passthrough  ExternalSaturationOutDataTypeStr=Inherit: Same as second input  aMode=0
  Control Roll : slpidlib/PID Controller  Controller=PID  Form=Parallel  TimeDomain=Continuous-time  UseExternalTs=off  SampleTime=-1  IntegratorMethod=Forward Euler  FilterMethod=Forward Euler  ControllerParametersSource=internal  P=attitude_kp  I=attitude_ki  UseKiTs=off  D=attitude_kd  N=attitude_f  UseFilter=on  TunerSelectOption=Transfer Function Based (PID Tuner App)  InitialConditionSource=internal  InitialConditionForIntegrator=0  InitialConditionForFilter=0  DifferentiatorICPrevScaledInput=0  ExternalReset=none  TrackingMode=off  Kt=1  LimitOutput=on  SatLimitsSource=internal  UpperSaturationLimit=attitude_limit  LowerSaturationLimit=-attitude_limit  LinearizeAsGain=on  AntiWindupMode=none  Kb=1  POutMin=[]  POutMax=[]  IOutMin=[]  IOutMax=[]  DOutMin=[]  DOutMax=[]  NOutMin=[]  NOutMax=[]  SumOutMin=[]  SumOutMax=[]  SaturationOutMin=[]  SaturationOutMax=[]  PParamMin=[]  PParamMax=[]  IParamMin=[]  IParamMax=[]  DParamMin=[]  DParamMax=[]  NParamMin=[]  NParamMax=[]  KbParamMin=[]  KbParamMax=[]  KtParamMin=[]  KtParamMax=[]  KbOutMin=[]  KbOutMax=[]  KtOutMin=[]  KtOutMax=[]  IntegratorOutMin=[]  IntegratorOutMax=[]  FilterOutMin=[]  FilterOutMax=[]  SumI1OutMin=[]  SumI1OutMax=[]  SumI2OutMin=[]  SumI2OutMax=[]  SumI3OutMin=[]  SumI3OutMax=[]  SumI4OutMin=[]  SumI4OutMax=[]  SumDOutMin=[]  SumDOutMax=[]  DifferentiatorOutMin=[]  DifferentiatorOutMax=[]  FilterDiffOutCoefMin=[]  FilterDiffOutCoefMax=[]  ReciprocalOutMin=[]  ReciprocalOutMax=[]  SumDenOutMin=[]  SumDenOutMax=[]  SumNumOutMin=[]  SumNumOutMax=[]  DivideOutMin=[]  DivideOutMax=[]  UdiffTsProdOutMin=[]  UdiffTsProdOutMax=[]  NTsProdOutMin=[]  NTsProdOutMax=[]  UintegralTsProdOutMin=[]  UintegralTsProdOutMax=[]  UngainTsProdOutMin=[]  UngainTsProdOutMax=[]  IntegratorContinuousStateAttributes=''  IntegratorStateMustResolveToSignalObject=off  IntegratorRTWStateStorageClass=Auto  FilterContinuousStateAttributes=''  FilterStateMustResolveToSignalObject=off  FilterRTWStateStorageClass=Auto  ParallelPVariant=InternalParameters  IdealPVariant=Disabled  IVariant=InternalParameters  DVariant=InternalParameters  IntegratorVariant=Continuous  SatVariant=Enabled  AWVariant=Passthrough  PCopyVariant=Disabled  TRVariant=Disabled  FdbkBlocksVariant=Forward  IdealPFdbkVariant=Disabled  SatFdbkVariant=Disabled  DerivativeFilterVariant=ContFilter  NVariant=InternalParameters  NCopyVariant=Disabled  FilterICVariant=InternalICsFilter  IntegratorICVariant=InternalICs  ExternalResetVariant=Disabled  TRSumVariant=Passthrough  SumFdbkVariant=Disabled  SumVariant=Sum_PID  TsampFilterVariant=InternalTs  TsampNgainVariant=Passthrough  TsampIntegralVariant=Passthrough  ExternalSaturationOutDataTypeStr=Inherit: Same as second input  aMode=0
  Control Thrust : slpidlib/PID Controller  Controller=PID  Form=Parallel  TimeDomain=Continuous-time  UseExternalTs=off  SampleTime=-1  IntegratorMethod=Forward Euler  FilterMethod=Forward Euler  ControllerParametersSource=internal  P=altitude_kp  I=altitude_ki  UseKiTs=off  D=altitude_kd  N=altitude_f  UseFilter=on  TunerSelectOption=Transfer Function Based (PID Tuner App)  ZeroCross=off  InitialConditionSource=internal  InitialConditionForIntegrator=0  InitialConditionForFilter=0  DifferentiatorICPrevScaledInput=0  ExternalReset=none  TrackingMode=off  Kt=1  LimitOutput=on  SatLimitsSource=internal  UpperSaturationLimit=altitude_limit  LowerSaturationLimit=-altitude_limit  LinearizeAsGain=on  AntiWindupMode=none  Kb=1  POutMin=[]  POutMax=[]  IOutMin=[]  IOutMax=[]  DOutMin=[]  DOutMax=[]  NOutMin=[]  NOutMax=[]  SumOutMin=[]  SumOutMax=[]  SaturationOutMin=[]  SaturationOutMax=[]  PParamMin=[]  PParamMax=[]  IParamMin=[]  IParamMax=[]  DParamMin=[]  DParamMax=[]  NParamMin=[]  NParamMax=[]  KbParamMin=[]  KbParamMax=[]  KtParamMin=[]  KtParamMax=[]  KbOutMin=[]  KbOutMax=[]  KtOutMin=[]  KtOutMax=[]  IntegratorOutMin=[]  IntegratorOutMax=[]  FilterOutMin=[]  FilterOutMax=[]  SumI1OutMin=[]  SumI1OutMax=[]  SumI2OutMin=[]  SumI2OutMax=[]  SumI3OutMin=[]  SumI3OutMax=[]  SumI4OutMin=[]  SumI4OutMax=[]  SumDOutMin=[]  SumDOutMax=[]  DifferentiatorOutMin=[]  DifferentiatorOutMax=[]  FilterDiffOutCoefMin=[]  FilterDiffOutCoefMax=[]  ReciprocalOutMin=[]  ReciprocalOutMax=[]  SumDenOutMin=[]  SumDenOutMax=[]  SumNumOutMin=[]  SumNumOutMax=[]  DivideOutMin=[]  DivideOutMax=[]  UdiffTsProdOutMin=[]  UdiffTsProdOutMax=[]  NTsProdOutMin=[]  NTsProdOutMax=[]  UintegralTsProdOutMin=[]  UintegralTsProdOutMax=[]  UngainTsProdOutMin=[]  UngainTsProdOutMax=[]  IntegratorContinuousStateAttributes=''  IntegratorStateMustResolveToSignalObject=off  IntegratorRTWStateStorageClass=Auto  FilterContinuousStateAttributes=''  FilterStateMustResolveToSignalObject=off  FilterRTWStateStorageClass=Auto  ParallelPVariant=InternalParameters  IdealPVariant=Disabled  IVariant=InternalParameters  DVariant=InternalParameters  IntegratorVariant=Continuous  SatVariant=Enabled  AWVariant=Passthrough  PCopyVariant=Disabled  TRVariant=Disabled  FdbkBlocksVariant=Forward  IdealPFdbkVariant=Disabled  SatFdbkVariant=Disabled  DerivativeFilterVariant=ContFilter  NVariant=InternalParameters  NCopyVariant=Disabled  FilterICVariant=InternalICsFilter  IntegratorICVariant=InternalICs  ExternalResetVariant=Disabled  TRSumVariant=Passthrough  SumFdbkVariant=Disabled  SumVariant=Sum_PID  TsampFilterVariant=InternalTs  TsampNgainVariant=Passthrough  TsampIntegralVariant=Passthrough  ExternalSaturationOutDataTypeStr=Inherit: Same as second input  aMode=0
  Control Yaw : slpidlib/PID Controller  Controller=PID  Form=Parallel  TimeDomain=Continuous-time  UseExternalTs=off  SampleTime=-1  IntegratorMethod=Forward Euler  FilterMethod=Forward Euler  ControllerParametersSource=internal  P=yaw_kp  I=yaw_ki  UseKiTs=off  D=yaw_kd  N=yaw_f  UseFilter=on  TunerSelectOption=Transfer Function Based (PID Tuner App)  InitialConditionSource=internal  InitialConditionForIntegrator=0  InitialConditionForFilter=0  DifferentiatorICPrevScaledInput=0  ExternalReset=none  TrackingMode=off  Kt=1  LimitOutput=on  SatLimitsSource=internal  UpperSaturationLimit=yaw_limit  LowerSaturationLimit=-yaw_limit  LinearizeAsGain=on  AntiWindupMode=none  Kb=1  POutMin=[]  POutMax=[]  IOutMin=[]  IOutMax=[]  DOutMin=[]  DOutMax=[]  NOutMin=[]  NOutMax=[]  SumOutMin=[]  SumOutMax=[]  SaturationOutMin=[]  SaturationOutMax=[]  PParamMin=[]  PParamMax=[]  IParamMin=[]  IParamMax=[]  DParamMin=[]  DParamMax=[]  NParamMin=[]  NParamMax=[]  KbParamMin=[]  KbParamMax=[]  KtParamMin=[]  KtParamMax=[]  KbOutMin=[]  KbOutMax=[]  KtOutMin=[]  KtOutMax=[]  IntegratorOutMin=[]  IntegratorOutMax=[]  FilterOutMin=[]  FilterOutMax=[]  SumI1OutMin=[]  SumI1OutMax=[]  SumI2OutMin=[]  SumI2OutMax=[]  SumI3OutMin=[]  SumI3OutMax=[]  SumI4OutMin=[]  SumI4OutMax=[]  SumDOutMin=[]  SumDOutMax=[]  DifferentiatorOutMin=[]  DifferentiatorOutMax=[]  FilterDiffOutCoefMin=[]  FilterDiffOutCoefMax=[]  ReciprocalOutMin=[]  ReciprocalOutMax=[]  SumDenOutMin=[]  SumDenOutMax=[]  SumNumOutMin=[]  SumNumOutMax=[]  DivideOutMin=[]  DivideOutMax=[]  UdiffTsProdOutMin=[]  UdiffTsProdOutMax=[]  NTsProdOutMin=[]  NTsProdOutMax=[]  UintegralTsProdOutMin=[]  UintegralTsProdOutMax=[]  UngainTsProdOutMin=[]  UngainTsProdOutMax=[]  IntegratorContinuousStateAttributes=''  IntegratorStateMustResolveToSignalObject=off  IntegratorRTWStateStorageClass=Auto  FilterContinuousStateAttributes=''  FilterStateMustResolveToSignalObject=off  FilterRTWStateStorageClass=Auto  ParallelPVariant=InternalParameters  IdealPVariant=Disabled  IVariant=InternalParameters  DVariant=InternalParameters  IntegratorVariant=Continuous  SatVariant=Enabled  AWVariant=Passthrough  PCopyVariant=Disabled  TRVariant=Disabled  FdbkBlocksVariant=Forward  IdealPFdbkVariant=Disabled  SatFdbkVariant=Disabled  DerivativeFilterVariant=ContFilter  NVariant=InternalParameters  NCopyVariant=Disabled  FilterICVariant=InternalICsFilter  IntegratorICVariant=InternalICs  ExternalResetVariant=Disabled  TRSumVariant=Passthrough  SumFdbkVariant=Disabled  SumVariant=Sum_PID  TsampFilterVariant=InternalTs  TsampNgainVariant=Passthrough  TsampIntegralVariant=Passthrough  ExternalSaturationOutDataTypeStr=Inherit: Same as second input  aMode=0
  Filter Pitch : TransferFcn  Denominator=[altitude_filtM 1]
  Filter Roll : TransferFcn  Denominator=[altitude_filtM 1]
  Filter Yaw : TransferFcn  Denominator=[yaw_filtM 1]
  Filter pz : TransferFcn  Denominator=[0.01 1]
  Gain4 : Gain  Gain=2*pi/(0.254^4 * sqrt(1.225))
  Mux : Mux  Inputs=2
  Mux1 : Mux  Inputs=2
  Pitch Control : Scope  NumInputPorts=3
  Select z : Selector  InputPortWidth=3  IndexOptions=Index vector (dialog)  Indices=[3]  OutputSizes=1
  Thrust Control : Scope  NumInputPorts=4
  Motor Pitch : Outport
  Motor Roll : Outport  Port=2
  Motor Yaw : Outport  Port=3
  Motor Thrust : Outport  Port=4
  wires:
  Roll Cmd/1 -> Add2/1
  Pitch Cmd/1 -> Mux1/1, Add7/1
  Add2/1 -> Control Roll/1
  In Bus Element3/1 -> Filter Yaw/1
  Add7/1 -> Pitch Control/2, Control Pitch/1
  Yaw Cmd/1 -> Add3/1
  In Bus Element2/1 -> Filter Pitch/1
  Select z/1 -> Mux/1, Add/1
  Control Pitch/1 -> Pitch Control/3, Motor Pitch/1
  In Bus Element1/1 -> Filter Roll/1
  Add3/1 -> Control Yaw/1
  Control Roll/1 -> Motor Roll/1
  In Bus Element9/1 -> Select z/1
  Add/1 -> Thrust Control/2, Control Thrust/1
  Control Thrust/1 -> Gain4/1, Thrust Control/3
  Mux/1 -> Thrust Control/1
  Gain4/1 -> Bias/1
  Mux1/1 -> Pitch Control/1
  Bias/1 -> Motor Thrust/1, Thrust Control/4
  Control Yaw/1 -> Motor Yaw/1
  In Bus Element4/1 -> Filter pz/1
  Filter Pitch/1 -> Mux1/2, Add7/2
  Filter Roll/1 -> Add2/2
  Filter Yaw/1 -> Add3/2
  Filter pz/1 -> Mux/2, Add/2

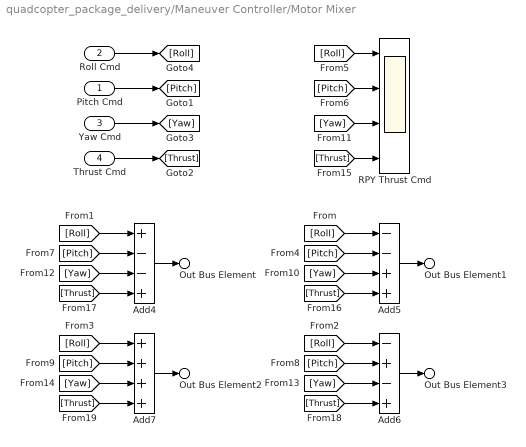
== system quadcopter_package_delivery/Maneuver Controller/Motor Mixer ==
  Pitch Cmd : Inport
  Roll Cmd : Inport  Port=2
  Yaw Cmd : Inport  Port=3
  Thrust Cmd : Inport  Port=4
  Add4 : Sum  Inputs=+--+
  Add5 : Sum  Inputs=--++
  Add6 : Sum  Inputs=-+-+
  Add7 : Sum  Inputs=++++
  RPY Thrust Cmd : Scope  NumInputPorts=4
  Out Bus Element : Outport  PortName=Cmd  Element=w1
  Out Bus Element1 : Outport  PortName=Cmd  Element=w2
  Out Bus Element2 : Outport  PortName=Cmd  Element=w3
  Out Bus Element3 : Outport  PortName=Cmd  Element=w4
  wires:
  Add7/1 -> Out Bus Element2/1
  Add6/1 -> Out Bus Element3/1
  Add4/1 -> Out Bus Element/1
  Add5/1 -> Out Bus Element1/1
  Roll Cmd/1 -> [Roll]
  Pitch Cmd/1 -> [Pitch]
  Yaw Cmd/1 -> [Yaw]
  Thrust Cmd/1 -> [Thrust]
  [Roll] -> Add5/1
  [Roll] -> Add4/1
  [Roll] -> Add6/1
  [Roll] -> Add7/1
  [Pitch] -> Add5/2
  [Roll] -> RPY Thrust Cmd/1
  [Pitch] -> RPY Thrust Cmd/2
  [Pitch] -> Add4/2
  [Pitch] -> Add6/2
  [Pitch] -> Add7/2
  [Yaw] -> Add5/3
  [Yaw] -> RPY Thrust Cmd/3
  [Yaw] -> Add4/3
  [Yaw] -> Add6/3
  [Yaw] -> Add7/3
  [Thrust] -> RPY Thrust Cmd/4
  [Thrust] -> Add5/4
  [Thrust] -> Add4/4
  [Thrust] -> Add6/4
  [Thrust] -> Add7/4

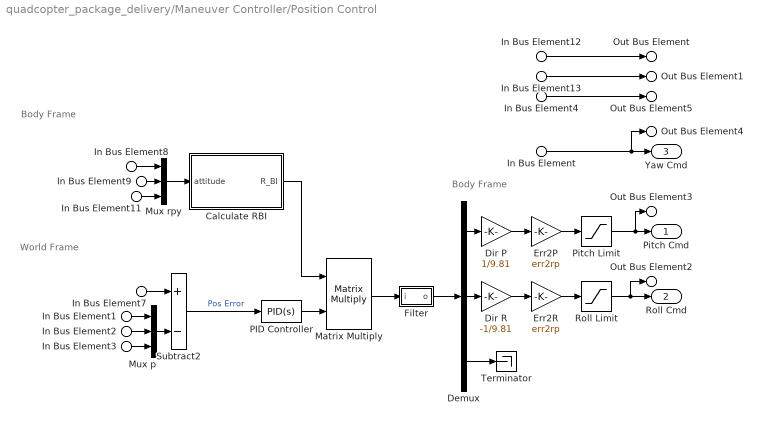
== system quadcopter_package_delivery/Maneuver Controller/Position Control ==
  note: Body Frame
  note: World Frame
  note: Body Frame
  In Bus Element1 : Inport  PortName=m  Element=Chassis.px
  In Bus Element2 : Inport  PortName=m  Element=Chassis.py
  In Bus Element3 : Inport  PortName=m  Element=Chassis.pz
  In Bus Element8 : Inport  PortName=m  Element=Chassis.roll
  In Bus Element9 : Inport  PortName=m  Element=Chassis.pitch
  In Bus Element11 : Inport  PortName=m  Element=Chassis.yaw
  In Bus Element7 : Inport  Port=2  PortName=Traj  Element=pos
  In Bus Element12 : Inport  Port=2  PortName=Traj  Element=pos
  In Bus Element13 : Inport  Port=2  PortName=Traj  Element=vel
  In Bus Element : Inport  Port=2  PortName=Traj  Element=yaw
  In Bus Element4 : Inport  Port=2  PortName=Traj  Element=acc
  Calculate RBI : MATLAB Function  TreatAsAtomicUnit=on
  Demux : Demux  Outputs=3
  Dir P : Gain  Gain=1/9.81
  Dir R : Gain  Gain=-1/9.81
  Err2P : Gain  Gain=err2rp
  Err2R : Gain  Gain=err2rp
  Filter : Subsystem  mask{filt_const=filt_pos4attitude}
      mask prompts: filt_const "Filter Constant"
  Matrix Multiply : Product  Multiplication=Matrix(*)
  Mux p : Mux  Inputs=3
  Mux rpy : Mux  Inputs=3
  PID Controller : slpidlib/PID Controller  Controller=PID  Form=Parallel  TimeDomain=Continuous-time  UseExternalTs=off  SampleTime=-1  IntegratorMethod=Forward Euler  FilterMethod=Forward Euler  ControllerParametersSource=internal  P=kp_xy2ypr  I=ki_xy2ypr  UseKiTs=off  D=kd_xy2ypr  N=filtD_xy2ypr  UseFilter=on  TunerSelectOption=Transfer Function Based (PID Tuner App)  InitialConditionSource=internal  InitialConditionForIntegrator=0  InitialConditionForFilter=0  DifferentiatorICPrevScaledInput=0  ExternalReset=none  TrackingMode=off  Kt=1  LimitOutput=off  SatLimitsSource=internal  UpperSaturationLimit=inf  LowerSaturationLimit=-inf  LinearizeAsGain=on  AntiWindupMode=none  Kb=1  POutMin=[]  POutMax=[]  IOutMin=[]  IOutMax=[]  DOutMin=[]  DOutMax=[]  NOutMin=[]  NOutMax=[]  SumOutMin=[]  SumOutMax=[]  SaturationOutMin=[]  SaturationOutMax=[]  PParamMin=[]  PParamMax=[]  IParamMin=[]  IParamMax=[]  DParamMin=[]  DParamMax=[]  NParamMin=[]  NParamMax=[]  KbParamMin=[]  KbParamMax=[]  KtParamMin=[]  KtParamMax=[]  KbOutMin=[]  KbOutMax=[]  KtOutMin=[]  KtOutMax=[]  IntegratorOutMin=[]  IntegratorOutMax=[]  FilterOutMin=[]  FilterOutMax=[]  SumI1OutMin=[]  SumI1OutMax=[]  SumI2OutMin=[]  SumI2OutMax=[]  SumI3OutMin=[]  SumI3OutMax=[]  SumI4OutMin=[]  SumI4OutMax=[]  SumDOutMin=[]  SumDOutMax=[]  DifferentiatorOutMin=[]  DifferentiatorOutMax=[]  FilterDiffOutCoefMin=[]  FilterDiffOutCoefMax=[]  ReciprocalOutMin=[]  ReciprocalOutMax=[]  SumDenOutMin=[]  SumDenOutMax=[]  SumNumOutMin=[]  SumNumOutMax=[]  DivideOutMin=[]  DivideOutMax=[]  UdiffTsProdOutMin=[]  UdiffTsProdOutMax=[]  NTsProdOutMin=[]  NTsProdOutMax=[]  UintegralTsProdOutMin=[]  UintegralTsProdOutMax=[]  UngainTsProdOutMin=[]  UngainTsProdOutMax=[]  IntegratorContinuousStateAttributes=''  IntegratorStateMustResolveToSignalObject=off  IntegratorRTWStateStorageClass=Auto  FilterContinuousStateAttributes=''  FilterStateMustResolveToSignalObject=off  FilterRTWStateStorageClass=Auto  ParallelPVariant=InternalParameters  IdealPVariant=Disabled  IVariant=InternalParameters  DVariant=InternalParameters  IntegratorVariant=Continuous  SatVariant=Disabled  AWVariant=Passthrough  PCopyVariant=Disabled  TRVariant=Disabled  FdbkBlocksVariant=Forward  IdealPFdbkVariant=Disabled  SatFdbkVariant=Disabled  DerivativeFilterVariant=ContFilter  NVariant=InternalParameters  NCopyVariant=Disabled  FilterICVariant=InternalICsFilter  IntegratorICVariant=InternalICs  ExternalResetVariant=Disabled  TRSumVariant=Passthrough  SumFdbkVariant=Disabled  SumVariant=Sum_PID  TsampFilterVariant=InternalTs  TsampNgainVariant=Passthrough  TsampIntegralVariant=Passthrough  ExternalSaturationOutDataTypeStr=Inherit: Same as second input  aMode=0
  Pitch Limit : Saturate  UpperLimit=pi/3  LowerLimit=-pi/3
  Roll Limit : Saturate  UpperLimit=pi/3  LowerLimit=-pi/3
  Subtract2 : Sum  Inputs=+-
  Terminator : Terminator
  Pitch Cmd : Outport
  Roll Cmd : Outport  Port=2
  Yaw Cmd : Outport  Port=3
  Out Bus Element : Outport  Port=4  PortName=Ref  Element=pos
  Out Bus Element1 : Outport  Port=4  PortName=Ref  Element=vel
  Out Bus Element2 : Outport  Port=4  PortName=Ref  Element=roll
  Out Bus Element3 : Outport  Port=4  PortName=Ref  Element=pitch
  Out Bus Element4 : Outport  Port=4  PortName=Ref  Element=yaw
  Out Bus Element5 : Outport  Port=4  PortName=Ref  Element=acc
  wires:
  Demux/2 -> Dir R/1
  Mux rpy/1 -> Calculate RBI/1(attitude)
  Demux/1 -> Dir P/1
  Calculate RBI/1(R_BI) -> Matrix Multiply/1
  Mux p/1 -> Subtract2/2
  Subtract2/1 -> PID Controller/1  "Pos Error"
  Err2R/1 -> Roll Limit/1
  In Bus Element7/1 -> Subtract2/1
  Err2P/1 -> Pitch Limit/1
  In Bus Element1/1 -> Mux p/1
  In Bus Element2/1 -> Mux p/2
  In Bus Element3/1 -> Mux p/3
  In Bus Element11/1 -> Mux rpy/3
  In Bus Element8/1 -> Mux rpy/1
  In Bus Element9/1 -> Mux rpy/2
  Pitch Limit/1 -> Out Bus Element3/1, Pitch Cmd/1
  Roll Limit/1 -> Out Bus Element2/1, Roll Cmd/1
  In Bus Element/1 -> Out Bus Element4/1, Yaw Cmd/1
  In Bus Element12/1 -> Out Bus Element/1
  In Bus Element13/1 -> Out Bus Element1/1
  PID Controller/1 -> Matrix Multiply/2
  Demux/3 -> Terminator/1
  Dir P/1 -> Err2P/1
  Dir R/1 -> Err2R/1
  Matrix Multiply/1 -> Filter/1(i)
  Filter/1(o) -> Demux/1
  In Bus Element4/1 -> Out Bus Element5/1
